simulink model "linear_model_fully_fault_sensor_non_linear"  (R2018b)
settings: Solver=VariableStepAuto  StartTime=0.0  StopTime=1000  RelTol=1e-3
values from neighbouring files (symbols this model uses):
  A11 = -pipeCoeff(1) * pipeCross(1) * sqrt(2*g) / (tankCross(1) * 2 * sqrt(Xe(1) - Xe(3)))    [ProblemData.m]
  A13 = -A11    [ProblemData.m]
  A22 = -pipeCoeff(2) * pipeCross(2) * sqrt(2*g) / (tankCross(2) * 2 * sqrt(Xe(3) - Xe(2))) - pipeCoeff(3) * pipeCross(3)* sqrt(2*g) / (tankCross(3) * 2 *sqrt(Xe(2)))    [ProblemData.m]
  A23 = pipeCoeff(2) * pipeCross(2) * sqrt(2*g) / (tankCross(2) * 2 * sqrt(Xe(3) - Xe(2)))    [ProblemData.m]
  A31 = pipeCoeff(1) * pipeCross(1) * sqrt(2*g) / (tankCross(3) * 2 * sqrt(Xe(1) - Xe(3)))    [ProblemData.m]
  A32 = pipeCoeff(2) * pipeCross(2) * sqrt(2*g) / (tankCross(3) * 2 * sqrt(Xe(3) - Xe(2)))    [ProblemData.m]
  A33 = -pipeCoeff(1) * pipeCross(1) * sqrt(2*g) / (tankCross(3) * 2 * sqrt(Xe(1) - Xe(3))) - pipeCoeff(2) * pipeCross(2) * sqrt(2*g) / (tankCross(3) * 2 * sqrt(Xe(3) - Xe(2)))    [ProblemData.m]
  B = [1/tankCross(1) 0 ... (first row only)    [ProblemData.m]
  faultMag = [0 0 0]    [ProblemData.m]
  faultTime = [1e6 1e6 1e6]    [ProblemData.m]
  K = place(A,B,p)'    [ProblemData.m]
  P = C * Cf' * (Cf * Cf')^-1    [ProblemData.m]
  pipeCoeff = [1 1 1]    [ProblemData.m]
  pipeCross = [5 5 5]*1e-4    [ProblemData.m]
  tankCross = [0.156 0.156 0.156]    [ProblemData.m]
  tankInit = [7 5 6]    [ProblemData.m]
  tankMax = [10 10 10]    [ProblemData.m]
  tankMin = [0 0 0]    [ProblemData.m]
  u0 = [1.5 2]*1e-3    [ProblemData.m]
  Xe = [7 5 6]    [ProblemData.m]
settings Model: Creator=TUDelft SID  LastModifiedBy=TUDelft SID

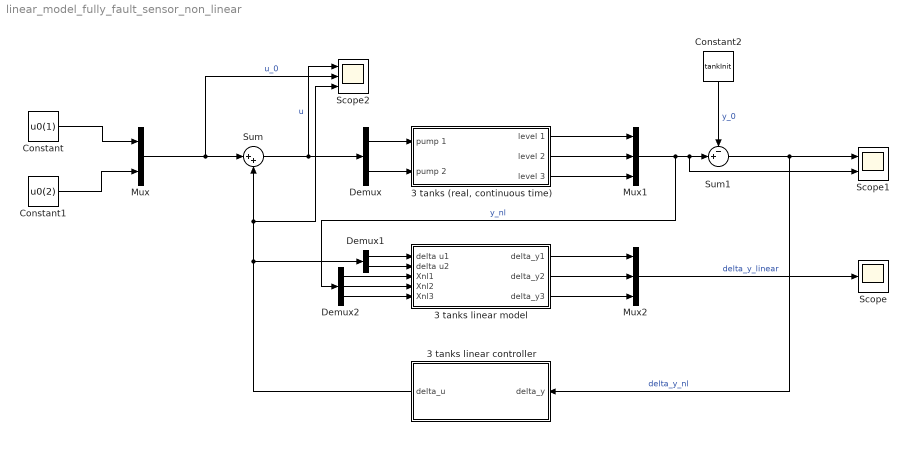
== system linear_model_fully_fault_sensor_non_linear ==
  "3 tanks (real, continuous time)" : Subsystem
  3 tanks linear controller : Subsystem
  3 tanks linear model : Subsystem
  Constant : Constant  Value=u0(1)
  Constant1 : Constant  Value=u0(2)
  Constant2 : Constant  Value=tankInit
  Demux : Demux  Outputs=2
  Demux1 : Demux  Outputs=2
  Demux2 : Demux  Outputs=3
  Mux : Mux  Inputs=2
  Mux1 : Mux  Inputs=3
  Mux2 : Mux  Inputs=3
  Scope : Scope
  Scope1 : Scope  NumInputPorts=2
  Scope2 : Scope  NumInputPorts=3
  Sum : Sum  Inputs=|++
  Sum1 : Sum  Inputs=-+|
  wires:
  Constant/1 -> Mux/1
  Constant1/1 -> Mux/2
  Demux/1 -> "3 tanks (real, continuous time)"/1(pump 1)
  Demux/2 -> "3 tanks (real, continuous time)"/2(pump 2)
  Sum/1 -> Demux/1, Scope2/1  "u"
  Mux/1 -> Scope2/2, Sum/1  "u_0"
  "3 tanks (real, continuous time)"/1(level 1) -> Mux1/1
  "3 tanks (real, continuous time)"/2(level 2) -> Mux1/2
  "3 tanks (real, continuous time)"/3(level 3) -> Mux1/3
  Mux1/1 -> Demux2/1, Scope1/2, Sum1/2  "y_nl"
  Constant2/1 -> Sum1/1  "y_0"
  3 tanks linear model/1(delta_y1) -> Mux2/1
  3 tanks linear controller/1(delta_u) -> Scope2/3, Sum/2, Demux1/1
  Mux2/1 -> Scope/1  "delta_y_linear"
  Demux2/3 -> 3 tanks linear model/5(Xnl3)
  Demux2/1 -> 3 tanks linear model/3(Xnl1)
  Sum1/1 -> 3 tanks linear controller/1(delta_y), Scope1/1  "delta_y_nl"
  3 tanks linear model/2(delta_y2) -> Mux2/2
  3 tanks linear model/3(delta_y3) -> Mux2/3
  Demux1/2 -> 3 tanks linear model/2(delta u2)
  Demux2/2 -> 3 tanks linear model/4(Xnl2)
  Demux1/1 -> 3 tanks linear model/1(delta u1)

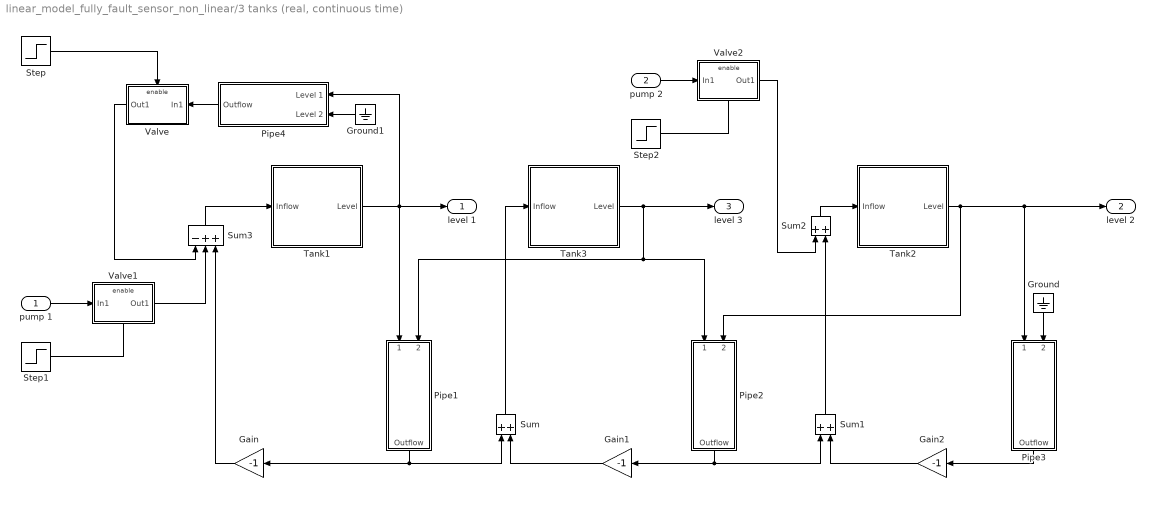
== system linear_model_fully_fault_sensor_non_linear/3 tanks (real, continuous time) ==
  pump 1 : Inport
  pump 2 : Inport  Port=2
  Gain : Gain  Gain=-1
  Gain1 : Gain  Gain=-1
  Gain2 : Gain  Gain=-1
  Ground : Ground
  Ground1 : Ground
  Pipe1 : Subsystem  mask(Connection Pipe){S_p=pipeCross(1), c_o=pipeCoeff(1)}
      mask prompts: S_p "Pipe cross-section [m^2]"; c_o "Outflow coefficient"
      mask help:
      | Connection pipe between two tanks.
      | The pipe cross-section and the outflow coefficient are mask block parameters.
      mask Help:
      | Enter the pipe cross-section [S_p] and the outflow coefficient [c_o] in the block dialog parameter fields.
      | 
      | The block generates the pipe's flow-rate. The input signals are the level of fluid into both the tanks, connected by the pipe. If the level in the first tank is bigger than the level in the second one, the fluid flow from the first to the second tank, else in the opposite way.
      mask Display: image(imread('pipe.jpg'));
  Pipe2 : Subsystem  mask(Connection Pipe){S_p=pipeCross(2), c_o=pipeCoeff(2)}
      mask prompts: S_p "Pipe cross-section [m^2]"; c_o "Outflow coefficient"
      mask help:
      | Connection pipe between two tanks.
      | The pipe cross-section and the outflow coefficient are mask block parameters.
      mask Help:
      | Enter the pipe cross-section [S_p] and the outflow coefficient [c_o] in the block dialog parameter fields.
      | 
      | The block generates the pipe's flow-rate. The input signals are the level of fluid into both the tanks, connected by the pipe. If the level in the first tank is bigger than the level in the second one, the fluid flow from the first to the second tank, else in the opposite way.
      mask Display: image(imread('pipe.jpg'));
  Pipe3 : Subsystem  mask(Connection Pipe){S_p=pipeCross(3), c_o=pipeCoeff(3)}
      mask prompts: S_p "Pipe cross-section [m^2]"; c_o "Outflow coefficient"
      mask help:
      | Connection pipe between two tanks.
      | The pipe cross-section and the outflow coefficient are mask block parameters.
      mask Help:
      | Enter the pipe cross-section [S_p] and the outflow coefficient [c_o] in the block dialog parameter fields.
      | 
      | The block generates the pipe's flow-rate. The input signals are the level of fluid into both the tanks, connected by the pipe. If the level in the first tank is bigger than the level in the second one, the fluid flow from the first to the second tank, else in the opposite way.
      mask Display: image(imread('pipe.jpg'));
  Pipe4 : Subsystem  mask(Connection Pipe){S_p=faultMag(2), c_o=1}
      mask prompts: S_p "Pipe cross-section [m^2]"; c_o "Outflow coefficient"
      mask help:
      | Connection pipe between two tanks.
      | The pipe cross-section and the outflow coefficient are mask block parameters.
      mask Help:
      | Enter the pipe cross-section [S_p] and the outflow coefficient [c_o] in the block dialog parameter fields.
      | 
      | The block generates the pipe's flow-rate. The input signals are the level of fluid into both the tanks, connected by the pipe. If the level in the first tank is bigger than the level in the second one, the fluid flow from the first to the second tank, else in the opposite way.
      mask Display: image(imread('pipe.jpg'));
  Step : Step  Time=faultTime(2)  SampleTime=0
  Step1 : Step  Time=faultTime(1)  Before=1  After=1-faultMag(1)  SampleTime=0
  Step2 : Step  Time=faultTime(3)  Before=1  After=1-faultMag(3)  SampleTime=0
  Sum : Sum
  Sum1 : Sum
  Sum2 : Sum
  Sum3 : Sum  Inputs=-++
  Tank1 : Subsystem  mask(Tank system){S=tankCross(1), x_0=tankInit(1), max_level=tankMax(1), min_level=tankMin(1)}
      mask prompts: S "Tank cross-section [m^2]"; x_0 "Initial fluid level [m"; max_level "Maximum fluid level [m]"; min_level "Minimum fluid level [m]"
      mask help:
      | Model of  a simple tank system. The input is a fluid flow-rate (may be positive or negative), the output is the fluid level in the tank.
      |
      | The tank cross-section, the initial, minimum and maximum fluid level are mask block parameters.
      mask Help:
      | Enter the tank cross-section, the initial, minimum, maximum fluid level in the block dialog parameter fields.
      | 
      | The block models a simple tank system. The input is the fluid flow-rate (positive or negative) that feeds the system; the output is the fluid level in the tank.
      mask Display: image(imread('tank.jpg'));
  Tank2 : Subsystem  mask(Tank system){S=tankCross(2), x_0=tankInit(2), max_level=tankMax(2), min_level=tankMin(2)}
      mask prompts: S "Tank cross-section [m^2]"; x_0 "Initial fluid level [m"; max_level "Maximum fluid level [m]"; min_level "Minimum fluid level [m]"
      mask help:
      | Model of  a simple tank system. The input is a fluid flow-rate (may be positive or negative), the output is the fluid level in the tank.
      |
      | The tank cross-section, the initial, minimum and maximum fluid level are mask block parameters.
      mask Help:
      | Enter the tank cross-section, the initial, minimum, maximum fluid level in the block dialog parameter fields.
      | 
      | The block models a simple tank system. The input is the fluid flow-rate (positive or negative) that feeds the system; the output is the fluid level in the tank.
      mask Display: image(imread('tank.jpg'));
  Tank3 : Subsystem  mask(Tank system){S=tankCross(3), x_0=tankInit(3), max_level=tankMax(3), min_level=tankMin(3)}
      mask prompts: S "Tank cross-section [m^2]"; x_0 "Initial fluid level [m"; max_level "Maximum fluid level [m]"; min_level "Minimum fluid level [m]"
      mask help:
      | Model of  a simple tank system. The input is a fluid flow-rate (may be positive or negative), the output is the fluid level in the tank.
      |
      | The tank cross-section, the initial, minimum and maximum fluid level are mask block parameters.
      mask Help:
      | Enter the tank cross-section, the initial, minimum, maximum fluid level in the block dialog parameter fields.
      | 
      | The block models a simple tank system. The input is the fluid flow-rate (positive or negative) that feeds the system; the output is the fluid level in the tank.
      mask Display: image(imread('tank.jpg'));
  Valve : Subsystem  TreatAsAtomicUnit=on  mask(Valve subsystem){}
      mask help: Model of a valve. When the control signal is greather then 0, the output is equal to the input. Otherwise, the output is 0.
      mask Display: image(imread('valve.jpg'))
  Valve1 : Subsystem  TreatAsAtomicUnit=on  mask(Valve subsystem){}
      mask help: Model of a valve. When the control signal is greather then 0, the output is equal to the input. Otherwise, the output is 0.
      mask Display: image(imread('valve.jpg'))
  Valve2 : Subsystem  TreatAsAtomicUnit=on  mask(Valve subsystem){}
      mask help: Model of a valve. When the control signal is greather then 0, the output is equal to the input. Otherwise, the output is 0.
      mask Display: image(imread('valve.jpg'))
  level 1 : Outport
  level 2 : Outport  Port=2
  level 3 : Outport  Port=3
  wires:
  Sum/1 -> Tank3/1(Inflow)
  Gain1/1 -> Sum/2
  Pipe2/1(Outflow) -> Sum1/1, Gain1/1
  Gain/1 -> Sum3/3
  Tank2/1(Level) -> level 2/1, Pipe3/1(Level 1), Pipe2/2(Level 2)
  Sum1/1 -> Sum2/2
  Gain2/1 -> Sum1/2
  Pipe3/1(Outflow) -> Gain2/1
  Tank1/1(Level) -> Pipe1/1(Level 1), Pipe4/1(Level 1), level 1/1
  Tank3/1(Level) -> level 3/1, Pipe2/1(Level 1), Pipe1/2(Level 2)
  Pipe1/1(Outflow) -> Gain/1, Sum/1
  Valve2/1(Out1) -> Sum2/1
  Sum2/1 -> Tank2/1(Inflow)
  Sum3/1 -> Tank1/1(Inflow)
  Ground/1 -> Pipe3/2(Level 2)
  Ground1/1 -> Pipe4/2(Level 2)
  Pipe4/1(Outflow) -> Valve/1(In1)
  Valve/1(Out1) -> Sum3/1
  Step/1 -> Valve/Enable
  pump 1/1 -> Valve1/1(In1)
  Valve1/1(Out1) -> Sum3/2
  Step1/1 -> Valve1/Enable
  Step2/1 -> Valve2/Enable
  pump 2/1 -> Valve2/1(In1)

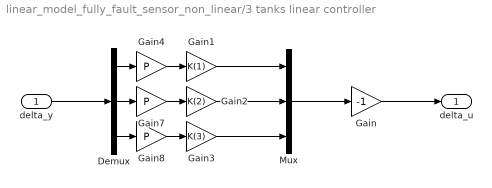
== system linear_model_fully_fault_sensor_non_linear/3 tanks linear controller ==
  delta_y : Inport
  Demux : Demux  Outputs=3
  Gain : Gain  Gain=-1
  Gain1 : Gain  Gain=K(1)
  Gain2 : Gain  Gain=K(2)
  Gain3 : Gain  Gain=K(3)
  Gain4 : Gain  Gain=P
  Gain7 : Gain  Gain=P
  Gain8 : Gain  Gain=P
  Mux : Mux  Inputs=3
  delta_u : Outport
  wires:
  Gain/1 -> delta_u/1
  delta_y/1 -> Demux/1
  Gain1/1 -> Mux/1
  Gain2/1 -> Mux/2
  Gain3/1 -> Mux/3
  Mux/1 -> Gain/1
  Demux/1 -> Gain4/1
  Gain4/1 -> Gain1/1
  Demux/2 -> Gain7/1
  Gain7/1 -> Gain2/1
  Demux/3 -> Gain8/1
  Gain8/1 -> Gain3/1

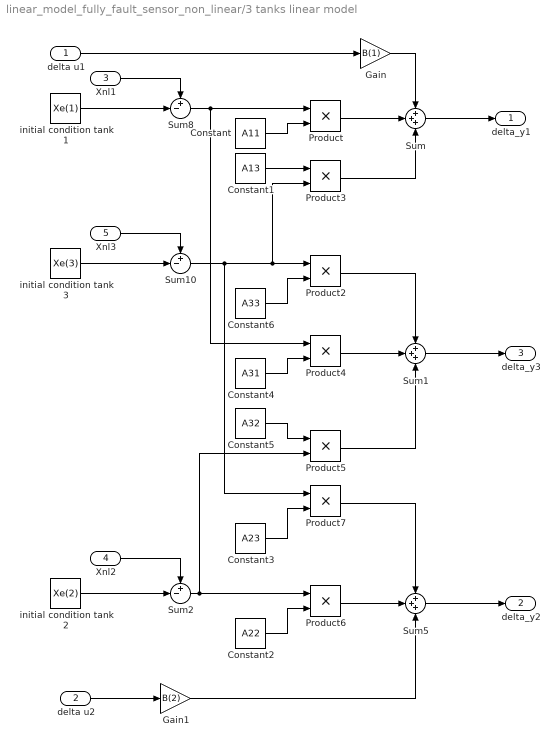
== system linear_model_fully_fault_sensor_non_linear/3 tanks linear model ==
  delta u1 : Inport
  delta u2 : Inport  Port=2
  Xnl1 : Inport  Port=3
  Xnl2 : Inport  Port=4
  Xnl3 : Inport  Port=5
  Constant : Constant  Value=A11
  Constant1 : Constant  Value=A13
  Constant2 : Constant  Value=A22
  Constant3 : Constant  Value=A23
  Constant4 : Constant  Value=A31
  Constant5 : Constant  Value=A32
  Constant6 : Constant  Value=A33
  Gain : Gain  Gain=B(1)
  Gain1 : Gain  Gain=B(2)
  Product{,2..7} (7 alike) : Product
  Sum : Sum  Inputs=+++
  Sum1 : Sum  Inputs=+++
  Sum10 : Sum  Inputs=+-|
  Sum2 : Sum  Inputs=+-|
  Sum5 : Sum  Inputs=+++
  Sum8 : Sum  Inputs=+-|
  initial condition tank 1 : Constant  Value=Xe(1)
  initial condition tank 2 : Constant  Value=Xe(2)
  initial condition tank 3 : Constant  Value=Xe(3)
  delta_y1 : Outport
  delta_y2 : Outport  Port=2
  delta_y3 : Outport  Port=3
  wires:
  delta u1/1 -> Gain/1
  Gain/1 -> Sum/1
  Sum/1 -> delta_y1/1
  Xnl1/1 -> Sum8/1
  Product/1 -> Sum/2
  Sum8/1 -> Product/1, Product4/1
  initial condition tank 1/1 -> Sum8/2
  Constant/1 -> Product/2
  Xnl3/1 -> Sum10/1
  initial condition tank 3/1 -> Sum10/2
  Sum10/1 -> Product7/1, Product3/2, Product2/1
  Constant1/1 -> Product3/1
  Product3/1 -> Sum/3
  Constant6/1 -> Product2/2
  Sum1/1 -> delta_y3/1
  Product2/1 -> Sum1/1
  Product4/1 -> Sum1/2
  Constant4/1 -> Product4/2
  Constant5/1 -> Product5/1
  Product5/1 -> Sum1/3
  initial condition tank 2/1 -> Sum2/2
  Xnl2/1 -> Sum2/1
  Sum2/1 -> Product5/2, Product6/1
  Constant2/1 -> Product6/2
  Product6/1 -> Sum5/2
  Sum5/1 -> delta_y2/1
  Product7/1 -> Sum5/1
  Constant3/1 -> Product7/2
  delta u2/1 -> Gain1/1
  Gain1/1 -> Sum5/3

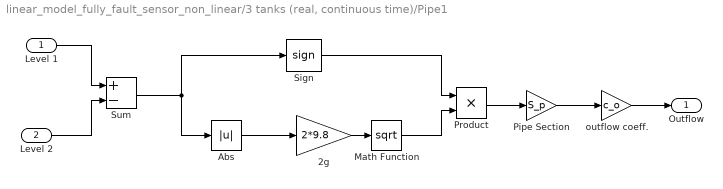
== system linear_model_fully_fault_sensor_non_linear/3 tanks (real, continuous time)/Pipe1 ==
  Level 1 : Inport
  Level 2 : Inport  Port=2
  2g : Gain  Gain=2*9.8  SaturateOnIntegerOverflow=on  OutDataTypeStr=Inherit: Same as input  ParamDataTypeStr=Inherit: Same as input
  Abs : Abs  SaturateOnIntegerOverflow=on
  Math Function : Math  Operator=sqrt  SaturateOnIntegerOverflow=on
  Pipe Section : Gain  Gain=S_p  SaturateOnIntegerOverflow=on  OutDataTypeStr=Inherit: Same as input  ParamDataTypeStr=Inherit: Same as input
  Product : Product  SaturateOnIntegerOverflow=on  InputSameDT=on  OutDataTypeStr=Inherit: Same as first input
  Sign : Signum
  Sum : Sum  Inputs=+-  SaturateOnIntegerOverflow=on  InputSameDT=on  OutDataTypeStr=Inherit: Same as first input
  outflow coeff. : Gain  Gain=c_o  SaturateOnIntegerOverflow=on  OutDataTypeStr=Inherit: Same as input  ParamDataTypeStr=Inherit: Same as input
  Outflow : Outport
  wires:
  outflow coeff./1 -> Outflow/1
  Pipe Section/1 -> outflow coeff./1
  Product/1 -> Pipe Section/1
  Sign/1 -> Product/1
  Math Function/1 -> Product/2
  2g/1 -> Math Function/1
  Abs/1 -> 2g/1
  Sum/1 -> Abs/1, Sign/1
  Level 2/1 -> Sum/2
  Level 1/1 -> Sum/1

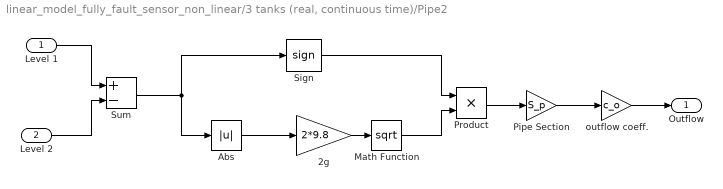
== system linear_model_fully_fault_sensor_non_linear/3 tanks (real, continuous time)/Pipe2 ==
  Level 1 : Inport
  Level 2 : Inport  Port=2
  2g : Gain  Gain=2*9.8  SaturateOnIntegerOverflow=on  OutDataTypeStr=Inherit: Same as input  ParamDataTypeStr=Inherit: Same as input
  Abs : Abs  SaturateOnIntegerOverflow=on
  Math Function : Math  Operator=sqrt  SaturateOnIntegerOverflow=on
  Pipe Section : Gain  Gain=S_p  SaturateOnIntegerOverflow=on  OutDataTypeStr=Inherit: Same as input  ParamDataTypeStr=Inherit: Same as input
  Product : Product  SaturateOnIntegerOverflow=on  InputSameDT=on  OutDataTypeStr=Inherit: Same as first input
  Sign : Signum
  Sum : Sum  Inputs=+-  SaturateOnIntegerOverflow=on  InputSameDT=on  OutDataTypeStr=Inherit: Same as first input
  outflow coeff. : Gain  Gain=c_o  SaturateOnIntegerOverflow=on  OutDataTypeStr=Inherit: Same as input  ParamDataTypeStr=Inherit: Same as input
  Outflow : Outport
  wires:
  outflow coeff./1 -> Outflow/1
  Pipe Section/1 -> outflow coeff./1
  Product/1 -> Pipe Section/1
  Sign/1 -> Product/1
  Math Function/1 -> Product/2
  2g/1 -> Math Function/1
  Abs/1 -> 2g/1
  Sum/1 -> Abs/1, Sign/1
  Level 2/1 -> Sum/2
  Level 1/1 -> Sum/1

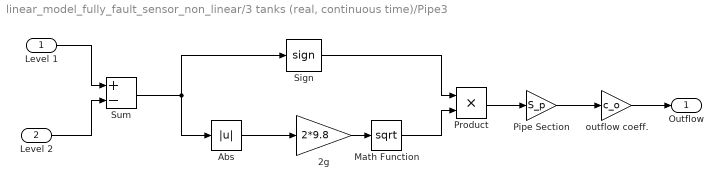
== system linear_model_fully_fault_sensor_non_linear/3 tanks (real, continuous time)/Pipe3 ==
  Level 1 : Inport
  Level 2 : Inport  Port=2
  2g : Gain  Gain=2*9.8  SaturateOnIntegerOverflow=on  OutDataTypeStr=Inherit: Same as input  ParamDataTypeStr=Inherit: Same as input
  Abs : Abs  SaturateOnIntegerOverflow=on
  Math Function : Math  Operator=sqrt  SaturateOnIntegerOverflow=on
  Pipe Section : Gain  Gain=S_p  SaturateOnIntegerOverflow=on  OutDataTypeStr=Inherit: Same as input  ParamDataTypeStr=Inherit: Same as input
  Product : Product  SaturateOnIntegerOverflow=on  InputSameDT=on  OutDataTypeStr=Inherit: Same as first input
  Sign : Signum
  Sum : Sum  Inputs=+-  SaturateOnIntegerOverflow=on  InputSameDT=on  OutDataTypeStr=Inherit: Same as first input
  outflow coeff. : Gain  Gain=c_o  SaturateOnIntegerOverflow=on  OutDataTypeStr=Inherit: Same as input  ParamDataTypeStr=Inherit: Same as input
  Outflow : Outport
  wires:
  outflow coeff./1 -> Outflow/1
  Pipe Section/1 -> outflow coeff./1
  Product/1 -> Pipe Section/1
  Sign/1 -> Product/1
  Math Function/1 -> Product/2
  2g/1 -> Math Function/1
  Abs/1 -> 2g/1
  Sum/1 -> Abs/1, Sign/1
  Level 2/1 -> Sum/2
  Level 1/1 -> Sum/1

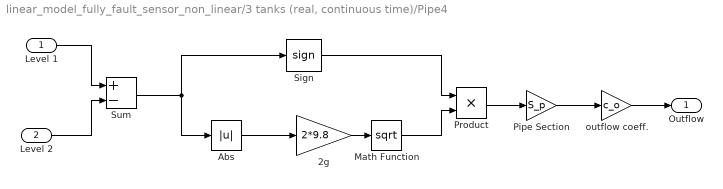
== system linear_model_fully_fault_sensor_non_linear/3 tanks (real, continuous time)/Pipe4 ==
  Level 1 : Inport
  Level 2 : Inport  Port=2
  2g : Gain  Gain=2*9.8  SaturateOnIntegerOverflow=on  OutDataTypeStr=Inherit: Same as input  ParamDataTypeStr=Inherit: Same as input
  Abs : Abs  SaturateOnIntegerOverflow=on
  Math Function : Math  Operator=sqrt  SaturateOnIntegerOverflow=on
  Pipe Section : Gain  Gain=S_p  SaturateOnIntegerOverflow=on  OutDataTypeStr=Inherit: Same as input  ParamDataTypeStr=Inherit: Same as input
  Product : Product  SaturateOnIntegerOverflow=on  InputSameDT=on  OutDataTypeStr=Inherit: Same as first input
  Sign : Signum
  Sum : Sum  Inputs=+-  SaturateOnIntegerOverflow=on  InputSameDT=on  OutDataTypeStr=Inherit: Same as first input
  outflow coeff. : Gain  Gain=c_o  SaturateOnIntegerOverflow=on  OutDataTypeStr=Inherit: Same as input  ParamDataTypeStr=Inherit: Same as input
  Outflow : Outport
  wires:
  outflow coeff./1 -> Outflow/1
  Pipe Section/1 -> outflow coeff./1
  Product/1 -> Pipe Section/1
  Sign/1 -> Product/1
  Math Function/1 -> Product/2
  2g/1 -> Math Function/1
  Abs/1 -> 2g/1
  Sum/1 -> Abs/1, Sign/1
  Level 2/1 -> Sum/2
  Level 1/1 -> Sum/1

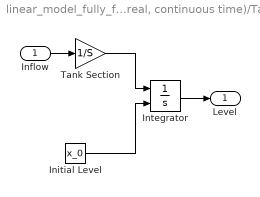
== system linear_model_fully_fault_sensor_non_linear/3 tanks (real, continuous time)/Tank1 ==
  Inflow : Inport
  Initial Level : Constant  Value=x_0
  Integrator : Integrator  InitialConditionSource=external  LimitOutput=on  UpperSaturationLimit=max_level  LowerSaturationLimit=min_level
  Tank Section : Gain  Gain=1/S  SaturateOnIntegerOverflow=on  OutDataTypeStr=Inherit: Same as input  ParamDataTypeStr=Inherit: Same as input
  Level : Outport  InitialOutput=0
  wires:
  Integrator/1 -> Level/1
  Initial Level/1 -> Integrator/2
  Tank Section/1 -> Integrator/1
  Inflow/1 -> Tank Section/1

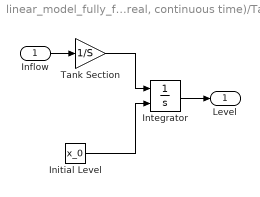
== system linear_model_fully_fault_sensor_non_linear/3 tanks (real, continuous time)/Tank2 ==
  Inflow : Inport
  Initial Level : Constant  Value=x_0
  Integrator : Integrator  InitialConditionSource=external  LimitOutput=on  UpperSaturationLimit=max_level  LowerSaturationLimit=min_level
  Tank Section : Gain  Gain=1/S  SaturateOnIntegerOverflow=on  OutDataTypeStr=Inherit: Same as input  ParamDataTypeStr=Inherit: Same as input
  Level : Outport  InitialOutput=0
  wires:
  Integrator/1 -> Level/1
  Initial Level/1 -> Integrator/2
  Tank Section/1 -> Integrator/1
  Inflow/1 -> Tank Section/1

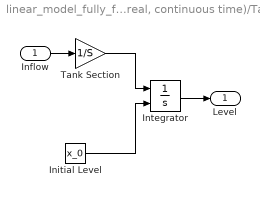
== system linear_model_fully_fault_sensor_non_linear/3 tanks (real, continuous time)/Tank3 ==
  Inflow : Inport
  Initial Level : Constant  Value=x_0
  Integrator : Integrator  InitialConditionSource=external  LimitOutput=on  UpperSaturationLimit=max_level  LowerSaturationLimit=min_level
  Tank Section : Gain  Gain=1/S  SaturateOnIntegerOverflow=on  OutDataTypeStr=Inherit: Same as input  ParamDataTypeStr=Inherit: Same as input
  Level : Outport  InitialOutput=0
  wires:
  Integrator/1 -> Level/1
  Initial Level/1 -> Integrator/2
  Tank Section/1 -> Integrator/1
  Inflow/1 -> Tank Section/1

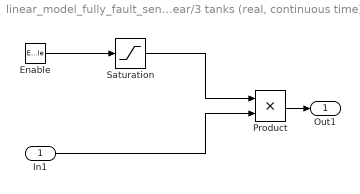
== system linear_model_fully_fault_sensor_non_linear/3 tanks (real, continuous time)/Valve ==
  In1 : Inport
  Enable : EnablePort  StatesWhenEnabling=reset  ShowOutputPort=on
  Product : Product  SaturateOnIntegerOverflow=on  InputSameDT=on  OutDataTypeStr=Inherit: Same as first input
  Saturation : Saturate  UpperLimit=1.0  LowerLimit=0.0
  Out1 : Outport  OutputWhenDisabled=reset  InitialOutput=0
  wires:
  Enable/1 -> Saturation/1
  Saturation/1 -> Product/1
  In1/1 -> Product/2
  Product/1 -> Out1/1

== system linear_model_fully_fault_sensor_non_linear/3 tanks (real, continuous time)/Valve1 ==
  In1 : Inport
  Enable : EnablePort  StatesWhenEnabling=reset  ShowOutputPort=on
  Product : Product  SaturateOnIntegerOverflow=on  InputSameDT=on  OutDataTypeStr=Inherit: Same as first input
  Saturation : Saturate  UpperLimit=1.0  LowerLimit=0.0
  Out1 : Outport  OutputWhenDisabled=reset  InitialOutput=0
  wires:
  Enable/1 -> Saturation/1
  Saturation/1 -> Product/1
  In1/1 -> Product/2
  Product/1 -> Out1/1

== system linear_model_fully_fault_sensor_non_linear/3 tanks (real, continuous time)/Valve2 ==
  In1 : Inport
  Enable : EnablePort  StatesWhenEnabling=reset  ShowOutputPort=on
  Product : Product  SaturateOnIntegerOverflow=on  InputSameDT=on  OutDataTypeStr=Inherit: Same as first input
  Saturation : Saturate  UpperLimit=1.0  LowerLimit=0.0
  Out1 : Outport  OutputWhenDisabled=reset  InitialOutput=0
  wires:
  Enable/1 -> Saturation/1
  Saturation/1 -> Product/1
  In1/1 -> Product/2
  Product/1 -> Out1/1
